simulink library "statesFileSimulinkLibObj"  (R2019a)
settings: Solver=VariableStepAuto  StartTime=0.0  StopTime=10.0  RelTol=1e-3
settings Model: Creator=agmotes  LastModifiedBy=agmotes

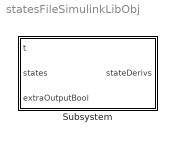
== system statesFileSimulinkLibObj ==
  Subsystem : Subsystem  mask{runfile=0, eqnsFile=0, stallFile=0}
      mask prompts: runfile "RunFileName"; eqnsFile "EqnsFileName"; stallFile "StallFileName"

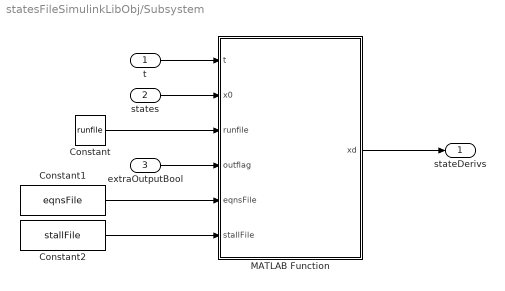
== system statesFileSimulinkLibObj/Subsystem ==
  t : Inport
  states : Inport  Port=2
  extraOutputBool : Inport  Port=3
  Constant : Constant  Value=runfile
  Constant1 : Constant  Value=eqnsFile
  Constant2 : Constant  Value=stallFile
  MATLAB Function : MATLAB Function  TreatAsAtomicUnit=on
  stateDerivs : Outport
  wires:
  MATLAB Function/1(xd) -> stateDerivs/1
  t/1 -> MATLAB Function/1(t)
  states/1 -> MATLAB Function/2(x0)
  extraOutputBool/1 -> MATLAB Function/4(outflag)
  Constant2/1 -> MATLAB Function/6(stallFile)
  Constant1/1 -> MATLAB Function/5(eqnsFile)
  Constant/1 -> MATLAB Function/3(runfile)

== matlab function statesFileSimulinkLibObj/Subsystem/MATLAB Function ==
  data: t input; xd output; x0 input; runfile input; outflag input; eqnsFile input; stallFile input
function xd  = statesFile(t, x0, runfile, outflag,eqnsFile,stallFile)
% [xd] = statesFile(t, x0, runfile, EQNS, OCBm, outflag) returns the 
% state derivatives xd for a given time t, state vector x0, and parameters 
% when outflag == 0. When outflag == 1, statesFile returns parameters
% calculated during the integration process. 
persistent EQNS OCBm OvBO_B F;
if t == 0
    [EQNS,OCBm,OvBO_B,F] = eqnsFileInit(eqnsFile,stallFile);
end

% error handle
if isnumeric(outflag) ~= 1
    error('outflag needs to be numeric.');
elseif abs(outflag) > 1
    error('outflag needs to be either 0 or 1.');
end

% load parameters
eval(runfile);

% load 
% ---------------------------------------------------------------
xBO = x0(1);    % ICS(1) = xBO m, sail position
yBO = x0(2);    % ICS(2) = yBO m, r_B/O_B 
zBO = x0(3);    % ICS(3) = zBO m, 
uBO = x0(4);    % ICS(4) = uBO m/s, 
vBO = x0(5);    % ICS(5) = vBO m/s, 
wBO = x0(6);    % ICS(6) = wBO m/s, 
tta = x0(7);    % ICS(7) = tta rad, roll angle
phi = x0(8);    % ICS(8) = phi rad, pitch angle
pzi = x0(9);    % ICS(9) = psi rad, yaw angle
p = x0(10);      % ICS(10) = p rad/s, roll rate
q = x0(11);      % ICS(11) = q rad/s, pitch rate
r = x0(12);      % ICS(12) = r rad/s, yaw rate

% load rotation matrices
% ---------------------------------------------------------------
% MATLAB uses single index notation for matrices by
% going down the first column, then second column, etc. Thus, the
% indices would be (for a 4x3 matrix):
% [1, 5, 9]
% [2, 6, 10]
% [3, 7, 11]
% [4, 8, 12]
OCB = NaN(3, 3);
% QCB = OCB;
O_V_BO_B = NaN(3, 1);
for i1 = 1:9
    OCB(i1) = eval(OCBm{i1});
    % QCB(i1) = eval(QCBm{i1});
    if i1 < 4
        O_V_BO_B(i1) = eval(OvBO_B{i1});
    end
end
BCO = transpose(OCB);
% BCQ = transpose(QCB);
% QCO = QCB*BCO;

% angles 
% ----------------------------------------------------------------
vrel_B = [0; 0; 0];
alfa = 0;
beta = 0;
v_inertial_O = [vinf_iO; vinf_jO; vinf_kO];     % m/s, inertial winds
vrel_B = BCO*v_inertial_O - O_V_BO_B;       % m/s, relative wind - old
% % alfa = atan2(vrel_B(3), -vrel_B(1));        % rad, alfa
% % beta = -atan2(vrel_B(2), -vrel_B(1));       % rad, beta 
% % alfa = atan2(vrel_B(3), vrel_B(1));           % rad, Edkin alpha 
% % beta = asin(vrel_B(2)/norm(vrel_B));          % rad, Edkin beta
% alfa = -atan2(vrel_B(3), vrel_B(1));
% beta = atan2(vrel_B(2), vrel_B(1));

alfa = atan2(vrel_B(3), vrel_B(1));
BCS = MakeMatrix('y', alfa);
SCB = transpose(BCS);
vrel_S = SCB*vrel_B;
beta = atan2(vrel_S(2), vrel_S(1));
WCS = MakeMatrix('z', beta);

% TO DO
% 3. Simulate to confirm operation wiht simple model
% 
% 4. Add in full blown aero model for a single linearized point
%   a. run AVL for known case 
%   b. add read in stabs file expressions and setup full aero model
%   c. simulate to confirm operation



% aero model
% ----------------------------------------------------------------
% stall model
% ASSUME:
%   1. stall is a decrease in lift and sideforce on the sail around a
%       critical alpha. This is modeled as an erf "rolloff" type of effect. 
%       Stall is continuous to prevent ode45 from freaking out.
%   2. stall is assumed to only degrade lift and side force. Drag is
%       assumed to still act and be large (to correct the sail). 
% stallterm = 1;
stallterm = F(alfa*180/pi);    % return the reduction in stall [0, 1] due 
% to stall of alpha. stall alpha is around 15 deg and transitons within 2
% degrees
% Only adds ~0.5s for a 10s simulation to use F()

% aero switch case
CL = 0;
CD = 0;
CY = 0;
Cl = 0;
Cm = 0;
Cn = 0;
switch aeromodel
    case 'none'
        % do nothing
        Maero_S = [0; 0; 0];
        Fax = 0;
        Fay = 0;
        Faz = 0;
        Faero_S = [Fax; Fay; Faz];
    case 'dumb'
        % % dumb aero model
        % Fax = 5;   % N, drag   
        Fax = 0;
        Fay = 0;
        Faz = 5;
        Maero_S = [0; 0; 0];
        Faero_S = [Fax; Fay; Faz];
    case 'abde'
        % simple aero model
        vrelB = norm(vrel_B);   % m/s, magnitude of relative wind
        q_Pa = 0.5*rho*vrelB*vrelB;
        CL = CLa*alfa + CLb*beta + CLd1*de;
        CD = CDvis + CL*CL/(pi*AR*e);
        CY = CYa*alfa + CYb*beta +CYd1*de;
        CL = CL*stallterm;
        CY = CY*stallterm;
        L = q_Pa*CL*Sref;
        D = q_Pa*CD*Sref;
        Y = q_Pa*CY*Sref;
        Faero_S = [D; Y; L];
        % moments
        Cl = Cla*alfa + Clb*beta + Cld1*de;
        Cm = Cma*alfa + Cmb*beta + Cmd1*de;
        Cn = Cna*alfa + Cnb*beta + Cnd1*de;
        l = q_Pa*Cl*Sref*b;
        m = q_Pa*Cm*Sref*c;
        n = q_Pa*Cn*Sref*b;
        Maero_S = [l; m; n];
    case 'abdepqr'
        % simple aero model
        vrelB = norm(vrel_B);   % m/s, magnitude of relative wind
        q_Pa = 0.5*rho*vrelB*vrelB;
        CL = CLa*alfa + CLb*beta + CLd1*de + CLp*p + CLq*q + CLr*r;
        CD = CDvis + CL*CL/(pi*AR*e);
        CY = CYa*alfa + CYb*beta +CYd1*de + CYp*p + CYq*q + CYr*r;
        CL = CL*stallterm;
        CY = CY*stallterm;
        L = q_Pa*CL*Sref;
        D = q_Pa*CD*Sref;
        Y = q_Pa*CY*Sref;
        Faero_S = [D; Y; L];
        % moments
        Cl = Cla*alfa + Clb*beta + Cld1*de + Clp*p + Clq*q + Clr*r;
        Cm = Cma*alfa + Cmb*beta + Cmd1*de + Cmp*p + Cmq*q + Cmr*r;
        Cn = Cna*alfa + Cnb*beta + Cnd1*de + Cnp*p + Cnq*q + Cnr*r;
        l = q_Pa*Cl*Sref*b;
        m = q_Pa*Cm*Sref*c;
        n = q_Pa*Cn*Sref*b;
        Maero_S = [l; m; n];
    otherwise
        error('aeromodel not specified.');
end
% SCB = transpose(BCS);
% SCW = transpose(WCS);


% % rotation from S to B frame is:
Faero_B = BCS*Faero_S;
Fax = Faero_B(1);
Fay = Faero_B(2);
Faz = Faero_B(3);
Maero_B = BCS*Maero_S;
Max = Maero_B(1);
May = Maero_B(2);
Maz = Maero_B(3);



% tension
% ----------------------------------------------------------------
% rGO_O = [0; L1; 0];
rGO_O = [0; 0; 0];      % for spherical pendulum model
rGO_B = BCO*rGO_O;
rBO_B = [xBO; yBO; zBO];
rPB_B = [xPB; yPB; 0];
rBP_B = -rPB_B;
% rBO = rBP + rPG + rGO 
% rBO - rBP - rGO = rPG
% rGP = - rBO + rBP + rGO
rGP_B = rBP_B + rGO_B - rBO_B;      % fixed for sphericla pendulum
OwB_B = [p; q; r];
OvBP_B = [0; 0; 0] + cross(OwB_B, rBP_B);
OvGO_B = [0; 0; 0] + cross(OwB_B, rGO_B); % fixed for spherical pendulum
OvBO_B = [uBO; vBO; wBO] + cross(OwB_B, rBO_B);
OvGP_B = OvBP_B + OvGO_B - OvBO_B;      % fixed for sphericla pendulum
% %   -> rBO - rBP - rGO = rPG 
% % rGP_B = rGO_B + rBP_B - rBO_B;
ds = max([norm(rGP_B) - L2, 0]);
% sign(ds) always either 0, or 1
% if ds = 0, min([+VE #, 0]) == 0 -> no stretch
% if ds = #, min([+VE #, 1e6]) == +VE # -> stretch!
% % dsd = min([norm(OvGP_B), sign(ds)*1e6]);  
% keyboard
% rGP -> tension is away from sail to balloon
% T_B = k*ds.*rGP_B/norm(rGP_B);
% T_B = (k*ds + ct*dsd).*rGP_B/norm(rGP_B)
% rGP_B(2)
% OvGP_B(2)
% k*ds.*rGP_B/norm(rGP_B)
% c*OvGP_B*sign(ds)
T_B = (k*ds).*rGP_B/norm(rGP_B) + ct*OvGP_B*sign(ds);
% OvGP_B(2)
dsd = OvGP_B(2);
% keyboard
% T_B = [0; 0; 0];
Tx = T_B(1);
Ty = T_B(2);
Tz = T_B(3);

% tension moment - post process calculation
MT_B = CrossMe(rPB_B, T_B);

% weight
% ---------------------------------------------------------------
W_O = [0; -MT*g; 0];
W_B = BCO*W_O;
Wx = W_B(1);
Wy = W_B(2);
Wz = W_B(3);



% equations
% ---------------------------------------------------------------
% u_dot, v_dot, w_dot, theta_dot, phi_dot, psi_dot, p_dot, q_dot, r_dot
xd = NaN(length(x0), 1);
xd(1:3) = [uBO; vBO; wBO];
for i1 = 1:9
    xd(i1 + 3) = eval(EQNS{i1});
end

% catch nan
if sum(isnan(xd)) > 0
    fprintf('Something is nan\n');
    keyboard
end

% handle output structures
if outflag == 1
    xdv = xd;
    xd = struct;
    xd.x0 = x0;
    xd.xdv = xdv;
    xd.Maero_B = [Max; May; Maz];
    xd.Faero_B = [Fax; Fay; Faz];
    xd.Tens_B = [Tx; Ty; Tz];
    xd.ds = ds;
    xd.BCO = BCO;
    xd.rGO_B = rGO_B;
    xd.rPB_B = rPB_B;
    xd.rGP_B = rGP_B;
    xd.alfa = alfa;
    xd.beta = beta;
    xd.runfile = runfile;
    xd.t = t;
    xd.vrel_B = vrel_B;
    xd.MT_B = MT_B;
    xd.coeffs = [CL; CD; CY];
    xd.momcoe = [Cl; Cm; Cn];
    xd.de = de;
    xd.stallterm = stallterm;
    xd.Tmag = norm(xd.Tens_B);
    xd.dsd = dsd;
end
